simulink model "SLDRT_test"  (R2024b)
settings: Solver=FixedStepAuto  StartTime=0.0  StopTime=inf  FixedStep=1E-1  RelTol=1e-3
libraries: instrumentlib x1
settings Model: Creator=abstract  LastModifiedBy=abstract

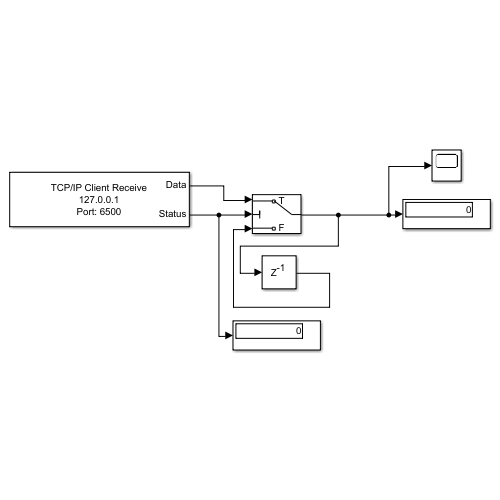
[thumbnail: Simulink's stored preview of the top-level diagram]
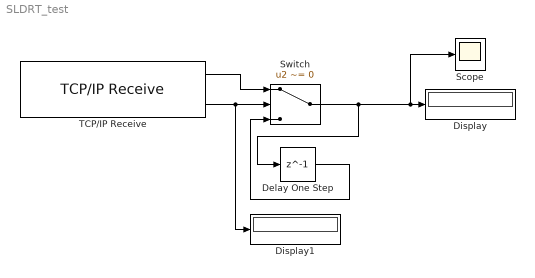
== system SLDRT_test ==
  Delay One Step : Delay  DelayLength=1
  Display : Display
  Display1 : Display
  Scope : Scope
  Switch : Switch  Criteria=u2 ~= 0  SaturateOnIntegerOverflow=off  InputSameDT=off
  TCP/IP Receive : instrumentlib/TCP//IP Receive  Host=127.0.0.1  Port=6500  DataSize=[1, 1]  DataType=ASCII  ASCIIFormatting=%d  Terminator=LF  CustomTerminator=10  ByteOrder=little-endian  EnableBlockingMode=off  Timeout=10  SampleTime=-1  SimulateUsing=Interpreted execution
  wires:
  Delay One Step/1 -> Switch/3
  TCP/IP Receive/1 -> Switch/1
  TCP/IP Receive/2 -> Display1/1, Switch/2
  Switch/1 -> Scope/1, Display/1, Delay One Step/1
